simulink subsystem "s0507_alpha_theta_PP_KF_polyfit"  (R2019b)
settings: Solver=VariableStepAuto  StartTime=0.0  StopTime=10.0  RelTol=1e-3
undefined symbols (not defined in the file): __PRM__SERIALIZED__DATA__, den_filter, Discrete, dt_control, num_filter, PARAMS, SubsystemReferenceBlock, Time
libraries: ctrlSharedLib x1
settings Model: Creator=paolo  LastModifiedBy=opc

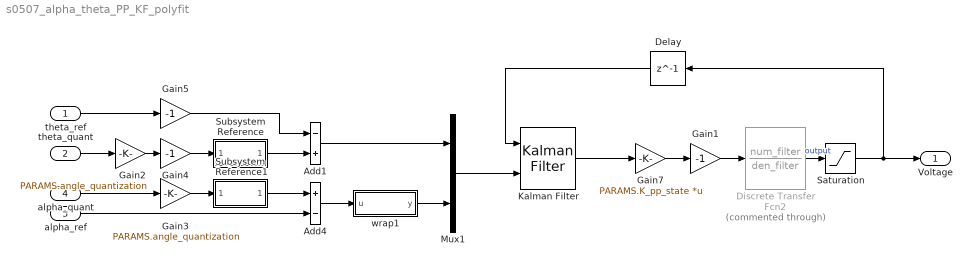
== system s0507_alpha_theta_PP_KF_polyfit ==
  theta_ref : Inport
  theta_quant : Inport  Port=2
  alpha_ref : Inport  Port=3
  alpha_quant : Inport  Port=4
  Add1 : Sum  Inputs=-+
  Add4 : Sum  Inputs=+-
  Delay : Delay  DelayLength=1
  Discrete Transfer Fcn2 : DiscreteTransferFcn  Commented=through  Numerator=num_filter  Denominator=den_filter  SampleTime=dt_control
  Gain1 : Gain  Gain=-1
  Gain2 : Gain  Gain=PARAMS.angle_quantization
  Gain3 : Gain  Gain=PARAMS.angle_quantization
  Gain4 : Gain  Gain=-1
  Gain5 : Gain  Gain=-1
  Gain7 : Gain  Gain=PARAMS.K_pp_state  Multiplication=Matrix(K*u)
  Kalman Filter : ctrlSharedLib/Kalman Filter  TimeDomain=Discrete-Time  UseCurrentEstimator=on  ModelSource=Individual A, B, C, D matrices  ModelSourceVariable=ss(0.95,1,1,0,1)  A=PARAMS.A_pi_DT  B=PARAMS.B_pi_DT  C=[1 0 0 0; 0 0 1 0]  D=[0; 0]  NumberOfStates=1  NumberOfInputs=1  NumberOfOutputs=1  InitialEstimateSource=Dialog  X0=[PARAMS.th_0, PARAMS.th_dot_0, 0, PARAMS.al_dot_0]  P0=10  UseK=off  UseGH=off  NumberOfProcessNoiseInputs=1  G=1  TimeInvariantG=on  H=0  TimeInvariantH=on  Q=diag([1, 1e9, 1, 1e9]);  TimeInvariantQ=on  R=diag([1e5, 1e5]);  TimeInvariantR=on  N=0  TimeInvariantN=on  AddInputPort=on  AddEnablePort=off  OutputEstimatedY=off  OutputP=off  Ts=-1
      settings: SourceProductBaseCode=CT
  Mux1 : Mux  Inputs=2
  Saturation : Saturate  UpperLimit=PARAMS.V_sat  LowerLimit=-PARAMS.V_sat
  Subsystem Reference : Subsystem  BlockKeywords=__PRM__SERIALIZED__DATA__:SubsystemReferenceBlock  ReferencedSubsystem=Polynomial_Filter
  Subsystem Reference1 : Subsystem  BlockKeywords=__PRM__SERIALIZED__DATA__:SubsystemReferenceBlock  ReferencedSubsystem=Polynomial_Filter
  wrap1 : MATLAB Function  TreatAsAtomicUnit=on
  Voltage : Outport
  wires:
  alpha_quant/1 -> Gain3/1
  Discrete Transfer Fcn2/1 -> Saturation/1  "output"
  Gain5/1 -> Add1/1
  theta_ref/1 -> Gain5/1
  Gain4/1 -> Subsystem Reference/1
  Gain1/1 -> Discrete Transfer Fcn2/1
  Saturation/1 -> Delay/1, Voltage/1
  Gain3/1 -> Subsystem Reference1/1
  Gain2/1 -> Gain4/1
  alpha_ref/1 -> Add4/2
  Gain7/1 -> Gain1/1
  theta_quant/1 -> Gain2/1
  Add4/1 -> wrap1/1(u)
  wrap1/1(y) -> Mux1/2
  Mux1/1 -> Kalman Filter/2
  Delay/1 -> Kalman Filter/1
  Add1/1 -> Mux1/1
  Kalman Filter/1 -> Gain7/1
  Subsystem Reference/1 -> Add1/2
  Subsystem Reference1/1 -> Add4/1

== matlab function s0507_alpha_theta_PP_KF_polyfit/wrap1 ==
  data: u input; y output
function y = wrap(u)
stop_condition = false;
y = u;
while ~stop_condition
    if y > pi
        y = y - 2*pi;
    elseif y < -pi
        y = y + 2*pi;
    else
        stop_condition = true;
    end
end
